simulink model "ERRH"  (R2025a)
settings: Solver=VariableStepAuto  StartTime=0.0  StopTime=5  MaxStep=1/50  RelTol=1e-3
settings Model: Creator=Szalay  LastModifiedBy=Szalay

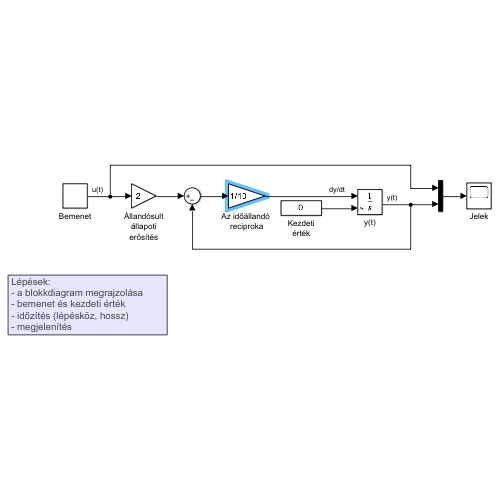
[thumbnail: Simulink's stored preview of the top-level diagram]
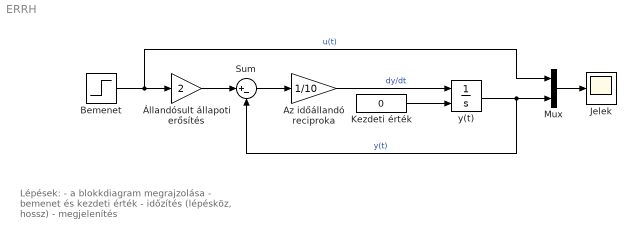
== system ERRH ==
  note: Lépések:
      | - a blokkdiagram megrajzolása
      | - bemenet és kezdeti érték
      | - időzítés (lépésköz, hossz)
      | - megjelenítés
  Az időállandó reciproka : Gain  Gain=1/10
  Bemenet : Step  Time=0  After=-2  SampleTime=0
  Jelek : Scope
      settings: ActiveDisplayYMinimum=-2.25  ActiveDisplayYMaximum=0.24999999999999994
  Kezdeti érték : Constant  Value=0
  Mux : Mux  Inputs=2
  Sum : Sum  Inputs=|+-
  y(t) : Integrator  InitialConditionSource=external
  Állandósult állapoti erősítés : Gain  Gain=2
  wires:
  Az időállandó reciproka/1 -> y(t)/1  "dy/dt"
  Sum/1 -> Az időállandó reciproka/1
  y(t)/1 -> Sum/2, Mux/2  "y(t)"
  Állandósult állapoti erősítés/1 -> Sum/1
  Bemenet/1 -> Mux/1, Állandósult állapoti erősítés/1  "u(t)"
  Kezdeti érték/1 -> y(t)/2
  Mux/1 -> Jelek/1
